simulink model "ScriptDemo"  (R2022b)
settings: configuration reference "TmVcThermal_Configuration_sub" (kept outside this file)
undefined symbols (not defined in the file): aaaa, bbbb, cTmComprCtrl_D_u8HvacFlowTable_db, cTmComprCtrl_D_u8HvacFlowTable_sw, cTmComprCtrl_n_i16ChillCmpIMax, cTmComprCtrl_n_i16ChillCmpIMin, cTmComprCtrl_n_i16ChillCmpIMin666, cTmComprCtrl_n_i16ChillCmpPMax, cTmComprCtrl_n_i16ChillCmpPMin, cTmComprCtrl_n_i16CmpChillCoolRpmKiMax, cTmComprCtrl_n_i16CmpChillCoolRpmKiMin, cTmComprCtrl_n_i16CmpChillCoolRpmKpMax, cTmComprCtrl_n_i16CmpChillCoolRpmKpMin, cTmComprCtrl_n_i16CmpCoolRpmKiMax, cTmComprCtrl_n_i16CmpCoolRpmKiMin, cTmComprCtrl_n_i16CmpCoolRpmKpMax, cTmComprCtrl_n_i16CmpCoolRpmKpMin, cTmComprCtrl_n_i16SM4CmpHeatKiMax, cTmComprCtrl_n_i16SM4CmpHeatKiMin, cTmComprCtrl_n_i16SM4CmpHeatKpMax, cTmComprCtrl_n_i16SM4CmpHeatKpMin, cTmComprCtrl_n_i16SM5CmpHeatKiMax, cTmComprCtrl_n_i16SM5CmpHeatKiMin, cTmComprCtrl_n_i16SM5CmpHeatKpMax, cTmComprCtrl_n_i16SM5CmpHeatKpMin, cTmComprCtrl_n_i16SM6CmpHeatKiMax, cTmComprCtrl_n_i16SM6CmpHeatKiMin, cTmComprCtrl_n_i16SM6CmpHeatKpMax, cTmComprCtrl_n_i16SM6CmpHeatKpMin, cTmComprCtrl_n_u16CmpMaxSpdFanFltLimt, cTmComprCtrl_n_u16CmpMaxSpdLoSidePFltLimt, cTmComprCtrl_n_u16CmpMaxSpdSensorFltLimt, cTmComprCtrl_n_u16CompMinRpm, cTmComprCtrl_n_u16CompRpmIncThres, cTmComprCtrl_t_u16BattCooltFFPeriod, cTmComprCtrl_t_u16BattCooltPIPeriod, cTmComprCtrl_t_u16CmpCoolFFPeriod, cTmComprCtrl_t_u16CmpCoolPIPeriod, cTmComprCtrl_t_u16CoolCmpChillFFPeriod, cTmComprCtrl_t_u16CoolCmpChillPIPeriod, cTmComprCtrl_t_u16SM4CmpHeatFFPeriod, cTmComprCtrl_t_u16SM4CmpHeatPIPeriod, cTmComprCtrl_t_u16SM5CmpHeatFFPeriod, cTmComprCtrl_t_u16SM5CmpHeatPIPeriod, cTmComprCtrl_t_u16SM6CmpHeatFFPeriod, cTmComprCtrl_t_u16SM6CmpHeatPIPeriod, cTmComprCtrl_Te_EvapClearInteg, cTmComprCtrl_Te_i16HpReqTempSaturoffset, cTmComprCtrl_Te_i16SatLpReplaceDiff, cTmComprCtrl_Te_i16SM3BatDiffStartEvapDecOffset, cTmComprCtrl_Te_i16SM3EvapLo, cTmComprCtrl_Te_i16SM3TBatDiffEntEvapDecOffset, cTmComprCtrl_Te_i16SM3TBatDiffEntEvapDecOffsetQuit, cTmComprCtrl_Te_s32ErrCmpChillPIContinueCoolH, cTmComprCtrl_Te_s32ErrCmpChillPIContinueCoolL, cTmComprCtrl_Te_s32ErrCmpPIContinueChillH, cTmComprCtrl_Te_s32ErrCmpPIContinueChillL, cTmComprCtrl_Te_s32ErrCmpPIContinueCoolH, cTmComprCtrl_Te_s32ErrCmpPIContinueCoolL, cTmComprCtrl_Te_s32ErrCmpPIContinueHeatH ... (+398)
libraries: simulink x782, PCMULib x640, simulink_need_slupdate x4
(part 10 of 41)

== system ScriptDemo/Create/Model/createModSig/After3 ==
  note: % 鼠标选中模型执行如下代码
      | createModSig(gcb,' testValue ',true)
  sTmRefriVlvCtrl_X_s32CEXVPosReqIn : Inport  OutDataTypeStr=single  OutputFunctionCall=on
  sTmRefriVlvCtrl_X_s32EEXVPosReqIn : Inport  Port=2  OutDataTypeStr=single
  sTmRefriVlvCtrl_X_s32BEXVPosReqIn : Inport  Port=3  OutDataTypeStr=single
  yTmRefriVlvCtrl_B_HpcCexvMovEnableIn : Inport  Port=4  OutDataTypeStr=boolean
  sTmRefriVlvCtrl_Z_u8CEXVInitStateIn : Inport  Port=5  OutDataTypeStr=uint8
  yTmRefriVlvCtrl_B_CexvCalibReqIn : Inport  Port=6  OutDataTypeStr=boolean
  yTmRefriVlvCtrl_B_HpcEexvMovEnableIn : Inport  Port=7  OutDataTypeStr=boolean
  sTmRefriVlvCtrl_Z_u8EEXVInitStateIn : Inport  Port=8  OutDataTypeStr=uint8
  yTmRefriVlvCtrl_B_EexvCalibReqIn : Inport  Port=9  OutDataTypeStr=boolean
  yTmRefriVlvCtrl_B_HpcBexvMovEnableIn : Inport  Port=10  OutDataTypeStr=boolean
  sTmRefriVlvCtrl_Z_u8BEXVInitStateIn : Inport  Port=11  OutDataTypeStr=uint8
  yTmRefriVlvCtrl_B_BexvCalibReqIn : Inport  Port=12  OutDataTypeStr=boolean
  sTmRefriVlvCtrl_X_s32SM3BexvMaxPosIn : Inport  Port=13  OutDataTypeStr=single
  yTmRefriVlvCtrl_B_EvapBattTLimBexvEnaIn : Inport  Port=14  OutDataTypeStr=boolean
  sTmRefriVlvCtrl_D_u8EexvRefriSwitchStIn : Inport  Port=15  OutDataTypeStr=uint8
  sTmRefriVlvCtrl_D_u8CexvRefriSwitchStIn : Inport  Port=16  OutDataTypeStr=uint8
  sTmRefriVlvCtrl_D_u8BexvRefriSwitchStIn : Inport  Port=17  OutDataTypeStr=uint8
  Before : Subsystem
  sTmRefriVlvCtrl_X_s32CEXVPosReq : Outport  OutDataTypeStr=single
  sTmRefriVlvCtrl_X_s32EEXVPosReq : Outport  Port=2  OutDataTypeStr=single
  sTmRefriVlvCtrl_X_s32BEXVPosReq : Outport  Port=3  OutDataTypeStr=single
  yTmRefriVlvCtrl_B_HpcCexvMovEnable : Outport  Port=4  OutDataTypeStr=boolean
  sTmRefriVlvCtrl_Z_u8CEXVInitState : Outport  Port=5  OutDataTypeStr=uint8
  yTmRefriVlvCtrl_B_CexvCalibReq : Outport  Port=6  OutDataTypeStr=boolean
  yTmRefriVlvCtrl_B_HpcEexvMovEnable : Outport  Port=7  OutDataTypeStr=boolean
  sTmRefriVlvCtrl_Z_u8EEXVInitState : Outport  Port=8  OutDataTypeStr=uint8
  yTmRefriVlvCtrl_B_EexvCalibReq : Outport  Port=9  OutDataTypeStr=boolean
  yTmRefriVlvCtrl_B_HpcBexvMovEnable : Outport  Port=10  OutDataTypeStr=boolean
  sTmRefriVlvCtrl_Z_u8BEXVInitState : Outport  Port=11  OutDataTypeStr=uint8
  yTmRefriVlvCtrl_B_BexvCalibReq : Outport  Port=12  OutDataTypeStr=boolean
  sTmRefriVlvCtrl_X_s32SM3BexvMaxPos : Outport  Port=13  OutDataTypeStr=single
  yTmRefriVlvCtrl_B_EvapBattTLimBexvEna : Outport  Port=14  OutDataTypeStr=boolean
  sTmRefriVlvCtrl_D_u8EexvRefriSwitchSt : Outport  Port=15  OutDataTypeStr=uint8
  sTmRefriVlvCtrl_D_u8CexvRefriSwitchSt : Outport  Port=16  OutDataTypeStr=uint8
  sTmRefriVlvCtrl_D_u8BexvRefriSwitchSt : Outport  Port=17  OutDataTypeStr=uint8
  wires:
  sTmRefriVlvCtrl_X_s32BEXVPosReqIn/1 -> Before/3(sTmRefriVlvCtrl_X_s32BEXVPosReqIn)  "sTmRefriVlvCtrl_X_s32BEXVPosReqIn"
  sTmRefriVlvCtrl_X_s32SM3BexvMaxPosIn/1 -> Before/13(sTmRefriVlvCtrl_X_s32SM3BexvMaxPosIn)  "sTmRefriVlvCtrl_X_s32SM3BexvMaxPosIn"
  sTmRefriVlvCtrl_Z_u8BEXVInitStateIn/1 -> Before/11(sTmRefriVlvCtrl_Z_u8BEXVInitStateIn)  "sTmRefriVlvCtrl_Z_u8BEXVInitStateIn"
  sTmRefriVlvCtrl_D_u8CexvRefriSwitchStIn/1 -> Before/16(sTmRefriVlvCtrl_D_u8CexvRefriSwitchStIn)  "sTmRefriVlvCtrl_D_u8CexvRefriSwitchStIn"
  yTmRefriVlvCtrl_B_EvapBattTLimBexvEnaIn/1 -> Before/14(yTmRefriVlvCtrl_B_EvapBattTLimBexvEnaIn)  "yTmRefriVlvCtrl_B_EvapBattTLimBexvEnaIn"
  yTmRefriVlvCtrl_B_HpcEexvMovEnableIn/1 -> Before/7(yTmRefriVlvCtrl_B_HpcEexvMovEnableIn)  "yTmRefriVlvCtrl_B_HpcEexvMovEnableIn"
  Before/3(sTmRefriVlvCtrl_X_s32BEXVPosReq) -> sTmRefriVlvCtrl_X_s32BEXVPosReq/1  "sTmRefriVlvCtrl_X_s32BEXVPosReq"
  yTmRefriVlvCtrl_B_EexvCalibReqIn/1 -> Before/9(yTmRefriVlvCtrl_B_EexvCalibReqIn)  "yTmRefriVlvCtrl_B_EexvCalibReqIn"
  Before/8(sTmRefriVlvCtrl_Z_u8EEXVInitState) -> sTmRefriVlvCtrl_Z_u8EEXVInitState/1  "sTmRefriVlvCtrl_Z_u8EEXVInitState"
  sTmRefriVlvCtrl_Z_u8EEXVInitStateIn/1 -> Before/8(sTmRefriVlvCtrl_Z_u8EEXVInitStateIn)  "sTmRefriVlvCtrl_Z_u8EEXVInitStateIn"
  yTmRefriVlvCtrl_B_HpcBexvMovEnableIn/1 -> Before/10(yTmRefriVlvCtrl_B_HpcBexvMovEnableIn)  "yTmRefriVlvCtrl_B_HpcBexvMovEnableIn"
  yTmRefriVlvCtrl_B_BexvCalibReqIn/1 -> Before/12(yTmRefriVlvCtrl_B_BexvCalibReqIn)  "yTmRefriVlvCtrl_B_BexvCalibReqIn"
  Before/5(sTmRefriVlvCtrl_Z_u8CEXVInitState) -> sTmRefriVlvCtrl_Z_u8CEXVInitState/1  "sTmRefriVlvCtrl_Z_u8CEXVInitState"
  Before/4(yTmRefriVlvCtrl_B_HpcCexvMovEnable) -> yTmRefriVlvCtrl_B_HpcCexvMovEnable/1  "yTmRefriVlvCtrl_B_HpcCexvMovEnable"
  Before/6(yTmRefriVlvCtrl_B_CexvCalibReq) -> yTmRefriVlvCtrl_B_CexvCalibReq/1  "yTmRefriVlvCtrl_B_CexvCalibReq"
  sTmRefriVlvCtrl_X_s32EEXVPosReqIn/1 -> Before/2(sTmRefriVlvCtrl_X_s32EEXVPosReqIn)  "sTmRefriVlvCtrl_X_s32EEXVPosReqIn"
  sTmRefriVlvCtrl_X_s32CEXVPosReqIn/1 -> Before/1(sTmRefriVlvCtrl_X_s32CEXVPosReqIn)  "sTmRefriVlvCtrl_X_s32CEXVPosReqIn"
  yTmRefriVlvCtrl_B_CexvCalibReqIn/1 -> Before/6(yTmRefriVlvCtrl_B_CexvCalibReqIn)  "yTmRefriVlvCtrl_B_CexvCalibReqIn"
  sTmRefriVlvCtrl_Z_u8CEXVInitStateIn/1 -> Before/5(sTmRefriVlvCtrl_Z_u8CEXVInitStateIn)  "sTmRefriVlvCtrl_Z_u8CEXVInitStateIn"
  yTmRefriVlvCtrl_B_HpcCexvMovEnableIn/1 -> Before/4(yTmRefriVlvCtrl_B_HpcCexvMovEnableIn)  "yTmRefriVlvCtrl_B_HpcCexvMovEnableIn"
  sTmRefriVlvCtrl_D_u8BexvRefriSwitchStIn/1 -> Before/17(sTmRefriVlvCtrl_D_u8BexvRefriSwitchStIn)  "sTmRefriVlvCtrl_D_u8BexvRefriSwitchStIn"
  Before/12(yTmRefriVlvCtrl_B_BexvCalibReq) -> yTmRefriVlvCtrl_B_BexvCalibReq/1  "yTmRefriVlvCtrl_B_BexvCalibReq"
  Before/11(sTmRefriVlvCtrl_Z_u8BEXVInitState) -> sTmRefriVlvCtrl_Z_u8BEXVInitState/1  "sTmRefriVlvCtrl_Z_u8BEXVInitState"
  Before/1(sTmRefriVlvCtrl_X_s32CEXVPosReq) -> sTmRefriVlvCtrl_X_s32CEXVPosReq/1  "sTmRefriVlvCtrl_X_s32CEXVPosReq"
  Before/7(yTmRefriVlvCtrl_B_HpcEexvMovEnable) -> yTmRefriVlvCtrl_B_HpcEexvMovEnable/1  "yTmRefriVlvCtrl_B_HpcEexvMovEnable"
  sTmRefriVlvCtrl_D_u8EexvRefriSwitchStIn/1 -> Before/15(sTmRefriVlvCtrl_D_u8EexvRefriSwitchStIn)  "sTmRefriVlvCtrl_D_u8EexvRefriSwitchStIn"
  Before/10(yTmRefriVlvCtrl_B_HpcBexvMovEnable) -> yTmRefriVlvCtrl_B_HpcBexvMovEnable/1  "yTmRefriVlvCtrl_B_HpcBexvMovEnable"
  Before/14(yTmRefriVlvCtrl_B_EvapBattTLimBexvEna) -> yTmRefriVlvCtrl_B_EvapBattTLimBexvEna/1  "yTmRefriVlvCtrl_B_EvapBattTLimBexvEna"
  Before/9(yTmRefriVlvCtrl_B_EexvCalibReq) -> yTmRefriVlvCtrl_B_EexvCalibReq/1  "yTmRefriVlvCtrl_B_EexvCalibReq"
  Before/15(sTmRefriVlvCtrl_D_u8EexvRefriSwitchSt) -> sTmRefriVlvCtrl_D_u8EexvRefriSwitchSt/1  "sTmRefriVlvCtrl_D_u8EexvRefriSwitchSt"
  Before/13(sTmRefriVlvCtrl_X_s32SM3BexvMaxPos) -> sTmRefriVlvCtrl_X_s32SM3BexvMaxPos/1  "sTmRefriVlvCtrl_X_s32SM3BexvMaxPos"
  Before/17(sTmRefriVlvCtrl_D_u8BexvRefriSwitchSt) -> sTmRefriVlvCtrl_D_u8BexvRefriSwitchSt/1  "sTmRefriVlvCtrl_D_u8BexvRefriSwitchSt"
  Before/2(sTmRefriVlvCtrl_X_s32EEXVPosReq) -> sTmRefriVlvCtrl_X_s32EEXVPosReq/1  "sTmRefriVlvCtrl_X_s32EEXVPosReq"
  Before/16(sTmRefriVlvCtrl_D_u8CexvRefriSwitchSt) -> sTmRefriVlvCtrl_D_u8CexvRefriSwitchSt/1  "sTmRefriVlvCtrl_D_u8CexvRefriSwitchSt"

== system ScriptDemo/Create/Model/createModSig/After4 ==
  note: % 鼠标选中模型执行如下代码
      | createModSig(gcb,' dispName ',true)
  sTmRefriVlvCtrl_X_s32CEXVPosReqIn : Inport  OutDataTypeStr=single  OutputFunctionCall=on
  sTmRefriVlvCtrl_X_s32EEXVPosReqIn : Inport  Port=2  OutDataTypeStr=single
  sTmRefriVlvCtrl_X_s32BEXVPosReqIn : Inport  Port=3  OutDataTypeStr=single
  yTmRefriVlvCtrl_B_HpcCexvMovEnableIn : Inport  Port=4  OutDataTypeStr=boolean
  sTmRefriVlvCtrl_Z_u8CEXVInitStateIn : Inport  Port=5  OutDataTypeStr=uint8
  yTmRefriVlvCtrl_B_CexvCalibReqIn : Inport  Port=6  OutDataTypeStr=boolean
  yTmRefriVlvCtrl_B_HpcEexvMovEnableIn : Inport  Port=7  OutDataTypeStr=boolean
  sTmRefriVlvCtrl_Z_u8EEXVInitStateIn : Inport  Port=8  OutDataTypeStr=uint8
  yTmRefriVlvCtrl_B_EexvCalibReqIn : Inport  Port=9  OutDataTypeStr=boolean
  yTmRefriVlvCtrl_B_HpcBexvMovEnableIn : Inport  Port=10  OutDataTypeStr=boolean
  sTmRefriVlvCtrl_Z_u8BEXVInitStateIn : Inport  Port=11  OutDataTypeStr=uint8
  yTmRefriVlvCtrl_B_BexvCalibReqIn : Inport  Port=12  OutDataTypeStr=boolean
  sTmRefriVlvCtrl_X_s32SM3BexvMaxPosIn : Inport  Port=13  OutDataTypeStr=single
  yTmRefriVlvCtrl_B_EvapBattTLimBexvEnaIn : Inport  Port=14  OutDataTypeStr=boolean
  sTmRefriVlvCtrl_D_u8EexvRefriSwitchStIn : Inport  Port=15  OutDataTypeStr=uint8
  sTmRefriVlvCtrl_D_u8CexvRefriSwitchStIn : Inport  Port=16  OutDataTypeStr=uint8
  sTmRefriVlvCtrl_D_u8BexvRefriSwitchStIn : Inport  Port=17  OutDataTypeStr=uint8
  Before : Subsystem
  sTmRefriVlvCtrl_X_s32CEXVPosReq : Outport  OutDataTypeStr=single
  sTmRefriVlvCtrl_X_s32EEXVPosReq : Outport  Port=2  OutDataTypeStr=single
  sTmRefriVlvCtrl_X_s32BEXVPosReq : Outport  Port=3  OutDataTypeStr=single
  yTmRefriVlvCtrl_B_HpcCexvMovEnable : Outport  Port=4  OutDataTypeStr=boolean
  sTmRefriVlvCtrl_Z_u8CEXVInitState : Outport  Port=5  OutDataTypeStr=uint8
  yTmRefriVlvCtrl_B_CexvCalibReq : Outport  Port=6  OutDataTypeStr=boolean
  yTmRefriVlvCtrl_B_HpcEexvMovEnable : Outport  Port=7  OutDataTypeStr=boolean
  sTmRefriVlvCtrl_Z_u8EEXVInitState : Outport  Port=8  OutDataTypeStr=uint8
  yTmRefriVlvCtrl_B_EexvCalibReq : Outport  Port=9  OutDataTypeStr=boolean
  yTmRefriVlvCtrl_B_HpcBexvMovEnable : Outport  Port=10  OutDataTypeStr=boolean
  sTmRefriVlvCtrl_Z_u8BEXVInitState : Outport  Port=11  OutDataTypeStr=uint8
  yTmRefriVlvCtrl_B_BexvCalibReq : Outport  Port=12  OutDataTypeStr=boolean
  sTmRefriVlvCtrl_X_s32SM3BexvMaxPos : Outport  Port=13  OutDataTypeStr=single
  yTmRefriVlvCtrl_B_EvapBattTLimBexvEna : Outport  Port=14  OutDataTypeStr=boolean
  sTmRefriVlvCtrl_D_u8EexvRefriSwitchSt : Outport  Port=15  OutDataTypeStr=uint8
  sTmRefriVlvCtrl_D_u8CexvRefriSwitchSt : Outport  Port=16  OutDataTypeStr=uint8
  sTmRefriVlvCtrl_D_u8BexvRefriSwitchSt : Outport  Port=17  OutDataTypeStr=uint8
  wires:
  sTmRefriVlvCtrl_X_s32BEXVPosReqIn/1 -> Before/3(sTmRefriVlvCtrl_X_s32BEXVPosReqIn)  "sTmRefriVlvCtrl_X_s32BEXVPosReqIn"
  sTmRefriVlvCtrl_X_s32SM3BexvMaxPosIn/1 -> Before/13(sTmRefriVlvCtrl_X_s32SM3BexvMaxPosIn)  "sTmRefriVlvCtrl_X_s32SM3BexvMaxPosIn"
  sTmRefriVlvCtrl_Z_u8BEXVInitStateIn/1 -> Before/11(sTmRefriVlvCtrl_Z_u8BEXVInitStateIn)  "sTmRefriVlvCtrl_Z_u8BEXVInitStateIn"
  sTmRefriVlvCtrl_D_u8CexvRefriSwitchStIn/1 -> Before/16(sTmRefriVlvCtrl_D_u8CexvRefriSwitchStIn)  "sTmRefriVlvCtrl_D_u8CexvRefriSwitchStIn"
  yTmRefriVlvCtrl_B_EvapBattTLimBexvEnaIn/1 -> Before/14(yTmRefriVlvCtrl_B_EvapBattTLimBexvEnaIn)  "yTmRefriVlvCtrl_B_EvapBattTLimBexvEnaIn"
  yTmRefriVlvCtrl_B_HpcEexvMovEnableIn/1 -> Before/7(yTmRefriVlvCtrl_B_HpcEexvMovEnableIn)  "yTmRefriVlvCtrl_B_HpcEexvMovEnableIn"
  Before/3(sTmRefriVlvCtrl_X_s32BEXVPosReq) -> sTmRefriVlvCtrl_X_s32BEXVPosReq/1  "sTmRefriVlvCtrl_X_s32BEXVPosReq"
  yTmRefriVlvCtrl_B_EexvCalibReqIn/1 -> Before/9(yTmRefriVlvCtrl_B_EexvCalibReqIn)  "yTmRefriVlvCtrl_B_EexvCalibReqIn"
  Before/8(sTmRefriVlvCtrl_Z_u8EEXVInitState) -> sTmRefriVlvCtrl_Z_u8EEXVInitState/1  "sTmRefriVlvCtrl_Z_u8EEXVInitState"
  sTmRefriVlvCtrl_Z_u8EEXVInitStateIn/1 -> Before/8(sTmRefriVlvCtrl_Z_u8EEXVInitStateIn)  "sTmRefriVlvCtrl_Z_u8EEXVInitStateIn"
  yTmRefriVlvCtrl_B_HpcBexvMovEnableIn/1 -> Before/10(yTmRefriVlvCtrl_B_HpcBexvMovEnableIn)  "yTmRefriVlvCtrl_B_HpcBexvMovEnableIn"
  yTmRefriVlvCtrl_B_BexvCalibReqIn/1 -> Before/12(yTmRefriVlvCtrl_B_BexvCalibReqIn)  "yTmRefriVlvCtrl_B_BexvCalibReqIn"
  Before/5(sTmRefriVlvCtrl_Z_u8CEXVInitState) -> sTmRefriVlvCtrl_Z_u8CEXVInitState/1  "sTmRefriVlvCtrl_Z_u8CEXVInitState"
  Before/4(yTmRefriVlvCtrl_B_HpcCexvMovEnable) -> yTmRefriVlvCtrl_B_HpcCexvMovEnable/1  "yTmRefriVlvCtrl_B_HpcCexvMovEnable"
  Before/6(yTmRefriVlvCtrl_B_CexvCalibReq) -> yTmRefriVlvCtrl_B_CexvCalibReq/1  "yTmRefriVlvCtrl_B_CexvCalibReq"
  sTmRefriVlvCtrl_X_s32EEXVPosReqIn/1 -> Before/2(sTmRefriVlvCtrl_X_s32EEXVPosReqIn)  "sTmRefriVlvCtrl_X_s32EEXVPosReqIn"
  sTmRefriVlvCtrl_X_s32CEXVPosReqIn/1 -> Before/1(sTmRefriVlvCtrl_X_s32CEXVPosReqIn)  "sTmRefriVlvCtrl_X_s32CEXVPosReqIn"
  yTmRefriVlvCtrl_B_CexvCalibReqIn/1 -> Before/6(yTmRefriVlvCtrl_B_CexvCalibReqIn)  "yTmRefriVlvCtrl_B_CexvCalibReqIn"
  sTmRefriVlvCtrl_Z_u8CEXVInitStateIn/1 -> Before/5(sTmRefriVlvCtrl_Z_u8CEXVInitStateIn)  "sTmRefriVlvCtrl_Z_u8CEXVInitStateIn"
  yTmRefriVlvCtrl_B_HpcCexvMovEnableIn/1 -> Before/4(yTmRefriVlvCtrl_B_HpcCexvMovEnableIn)  "yTmRefriVlvCtrl_B_HpcCexvMovEnableIn"
  sTmRefriVlvCtrl_D_u8BexvRefriSwitchStIn/1 -> Before/17(sTmRefriVlvCtrl_D_u8BexvRefriSwitchStIn)  "sTmRefriVlvCtrl_D_u8BexvRefriSwitchStIn"
  Before/12(yTmRefriVlvCtrl_B_BexvCalibReq) -> yTmRefriVlvCtrl_B_BexvCalibReq/1  "yTmRefriVlvCtrl_B_BexvCalibReq"
  Before/11(sTmRefriVlvCtrl_Z_u8BEXVInitState) -> sTmRefriVlvCtrl_Z_u8BEXVInitState/1  "sTmRefriVlvCtrl_Z_u8BEXVInitState"
  Before/1(sTmRefriVlvCtrl_X_s32CEXVPosReq) -> sTmRefriVlvCtrl_X_s32CEXVPosReq/1  "sTmRefriVlvCtrl_X_s32CEXVPosReq"
  Before/7(yTmRefriVlvCtrl_B_HpcEexvMovEnable) -> yTmRefriVlvCtrl_B_HpcEexvMovEnable/1  "yTmRefriVlvCtrl_B_HpcEexvMovEnable"
  sTmRefriVlvCtrl_D_u8EexvRefriSwitchStIn/1 -> Before/15(sTmRefriVlvCtrl_D_u8EexvRefriSwitchStIn)  "sTmRefriVlvCtrl_D_u8EexvRefriSwitchStIn"
  Before/10(yTmRefriVlvCtrl_B_HpcBexvMovEnable) -> yTmRefriVlvCtrl_B_HpcBexvMovEnable/1  "yTmRefriVlvCtrl_B_HpcBexvMovEnable"
  Before/14(yTmRefriVlvCtrl_B_EvapBattTLimBexvEna) -> yTmRefriVlvCtrl_B_EvapBattTLimBexvEna/1  "yTmRefriVlvCtrl_B_EvapBattTLimBexvEna"
  Before/9(yTmRefriVlvCtrl_B_EexvCalibReq) -> yTmRefriVlvCtrl_B_EexvCalibReq/1  "yTmRefriVlvCtrl_B_EexvCalibReq"
  Before/15(sTmRefriVlvCtrl_D_u8EexvRefriSwitchSt) -> sTmRefriVlvCtrl_D_u8EexvRefriSwitchSt/1  "sTmRefriVlvCtrl_D_u8EexvRefriSwitchSt"
  Before/13(sTmRefriVlvCtrl_X_s32SM3BexvMaxPos) -> sTmRefriVlvCtrl_X_s32SM3BexvMaxPos/1  "sTmRefriVlvCtrl_X_s32SM3BexvMaxPos"
  Before/17(sTmRefriVlvCtrl_D_u8BexvRefriSwitchSt) -> sTmRefriVlvCtrl_D_u8BexvRefriSwitchSt/1  "sTmRefriVlvCtrl_D_u8BexvRefriSwitchSt"
  Before/2(sTmRefriVlvCtrl_X_s32EEXVPosReq) -> sTmRefriVlvCtrl_X_s32EEXVPosReq/1  "sTmRefriVlvCtrl_X_s32EEXVPosReq"
  Before/16(sTmRefriVlvCtrl_D_u8CexvRefriSwitchSt) -> sTmRefriVlvCtrl_D_u8CexvRefriSwitchSt/1  "sTmRefriVlvCtrl_D_u8CexvRefriSwitchSt"

== system ScriptDemo/Create/Model/createModSig/Before ==
  sTmRefriVlvCtrl_X_s32CEXVPosReqIn : Inport  OutDataTypeStr=single  OutputFunctionCall=on
  sTmRefriVlvCtrl_X_s32EEXVPosReqIn : Inport  Port=2  OutDataTypeStr=single
  sTmRefriVlvCtrl_X_s32BEXVPosReqIn : Inport  Port=3  OutDataTypeStr=single
  yTmRefriVlvCtrl_B_HpcCexvMovEnableIn : Inport  Port=4  OutDataTypeStr=boolean
  sTmRefriVlvCtrl_Z_u8CEXVInitStateIn : Inport  Port=5  OutDataTypeStr=uint8
  yTmRefriVlvCtrl_B_CexvCalibReqIn : Inport  Port=6  OutDataTypeStr=boolean
  yTmRefriVlvCtrl_B_HpcEexvMovEnableIn : Inport  Port=7  OutDataTypeStr=boolean
  sTmRefriVlvCtrl_Z_u8EEXVInitStateIn : Inport  Port=8  OutDataTypeStr=uint8
  yTmRefriVlvCtrl_B_EexvCalibReqIn : Inport  Port=9  OutDataTypeStr=boolean
  yTmRefriVlvCtrl_B_HpcBexvMovEnableIn : Inport  Port=10  OutDataTypeStr=boolean
  sTmRefriVlvCtrl_Z_u8BEXVInitStateIn : Inport  Port=11  OutDataTypeStr=uint8
  yTmRefriVlvCtrl_B_BexvCalibReqIn : Inport  Port=12  OutDataTypeStr=boolean
  sTmRefriVlvCtrl_X_s32SM3BexvMaxPosIn : Inport  Port=13  OutDataTypeStr=single
  yTmRefriVlvCtrl_B_EvapBattTLimBexvEnaIn : Inport  Port=14  OutDataTypeStr=boolean
  sTmRefriVlvCtrl_D_u8EexvRefriSwitchStIn : Inport  Port=15  OutDataTypeStr=uint8
  sTmRefriVlvCtrl_D_u8CexvRefriSwitchStIn : Inport  Port=16  OutDataTypeStr=uint8
  sTmRefriVlvCtrl_D_u8BexvRefriSwitchStIn : Inport  Port=17  OutDataTypeStr=uint8
  Before : Subsystem
  sTmRefriVlvCtrl_X_s32CEXVPosReq : Outport  OutDataTypeStr=single
  sTmRefriVlvCtrl_X_s32EEXVPosReq : Outport  Port=2  OutDataTypeStr=single
  sTmRefriVlvCtrl_X_s32BEXVPosReq : Outport  Port=3  OutDataTypeStr=single
  yTmRefriVlvCtrl_B_HpcCexvMovEnable : Outport  Port=4  OutDataTypeStr=boolean
  sTmRefriVlvCtrl_Z_u8CEXVInitState : Outport  Port=5  OutDataTypeStr=uint8
  yTmRefriVlvCtrl_B_CexvCalibReq : Outport  Port=6  OutDataTypeStr=boolean
  yTmRefriVlvCtrl_B_HpcEexvMovEnable : Outport  Port=7  OutDataTypeStr=boolean
  sTmRefriVlvCtrl_Z_u8EEXVInitState : Outport  Port=8  OutDataTypeStr=uint8
  yTmRefriVlvCtrl_B_EexvCalibReq : Outport  Port=9  OutDataTypeStr=boolean
  yTmRefriVlvCtrl_B_HpcBexvMovEnable : Outport  Port=10  OutDataTypeStr=boolean
  sTmRefriVlvCtrl_Z_u8BEXVInitState : Outport  Port=11  OutDataTypeStr=uint8
  yTmRefriVlvCtrl_B_BexvCalibReq : Outport  Port=12  OutDataTypeStr=boolean
  sTmRefriVlvCtrl_X_s32SM3BexvMaxPos : Outport  Port=13  OutDataTypeStr=single
  yTmRefriVlvCtrl_B_EvapBattTLimBexvEna : Outport  Port=14  OutDataTypeStr=boolean
  sTmRefriVlvCtrl_D_u8EexvRefriSwitchSt : Outport  Port=15  OutDataTypeStr=uint8
  sTmRefriVlvCtrl_D_u8CexvRefriSwitchSt : Outport  Port=16  OutDataTypeStr=uint8
  sTmRefriVlvCtrl_D_u8BexvRefriSwitchSt : Outport  Port=17  OutDataTypeStr=uint8
  wires:
  sTmRefriVlvCtrl_X_s32CEXVPosReqIn/1 -> Before/1(sTmRefriVlvCtrl_X_s32CEXVPosReqIn)
  sTmRefriVlvCtrl_X_s32EEXVPosReqIn/1 -> Before/2(sTmRefriVlvCtrl_X_s32EEXVPosReqIn)
  sTmRefriVlvCtrl_X_s32BEXVPosReqIn/1 -> Before/3(sTmRefriVlvCtrl_X_s32BEXVPosReqIn)
  yTmRefriVlvCtrl_B_HpcCexvMovEnableIn/1 -> Before/4(yTmRefriVlvCtrl_B_HpcCexvMovEnableIn)
  sTmRefriVlvCtrl_Z_u8CEXVInitStateIn/1 -> Before/5(sTmRefriVlvCtrl_Z_u8CEXVInitStateIn)
  yTmRefriVlvCtrl_B_CexvCalibReqIn/1 -> Before/6(yTmRefriVlvCtrl_B_CexvCalibReqIn)
  yTmRefriVlvCtrl_B_HpcEexvMovEnableIn/1 -> Before/7(yTmRefriVlvCtrl_B_HpcEexvMovEnableIn)
  sTmRefriVlvCtrl_Z_u8EEXVInitStateIn/1 -> Before/8(sTmRefriVlvCtrl_Z_u8EEXVInitStateIn)
  yTmRefriVlvCtrl_B_EexvCalibReqIn/1 -> Before/9(yTmRefriVlvCtrl_B_EexvCalibReqIn)
  yTmRefriVlvCtrl_B_HpcBexvMovEnableIn/1 -> Before/10(yTmRefriVlvCtrl_B_HpcBexvMovEnableIn)
  sTmRefriVlvCtrl_Z_u8BEXVInitStateIn/1 -> Before/11(sTmRefriVlvCtrl_Z_u8BEXVInitStateIn)
  yTmRefriVlvCtrl_B_BexvCalibReqIn/1 -> Before/12(yTmRefriVlvCtrl_B_BexvCalibReqIn)
  sTmRefriVlvCtrl_X_s32SM3BexvMaxPosIn/1 -> Before/13(sTmRefriVlvCtrl_X_s32SM3BexvMaxPosIn)
  yTmRefriVlvCtrl_B_EvapBattTLimBexvEnaIn/1 -> Before/14(yTmRefriVlvCtrl_B_EvapBattTLimBexvEnaIn)
  sTmRefriVlvCtrl_D_u8EexvRefriSwitchStIn/1 -> Before/15(sTmRefriVlvCtrl_D_u8EexvRefriSwitchStIn)
  sTmRefriVlvCtrl_D_u8CexvRefriSwitchStIn/1 -> Before/16(sTmRefriVlvCtrl_D_u8CexvRefriSwitchStIn)
  sTmRefriVlvCtrl_D_u8BexvRefriSwitchStIn/1 -> Before/17(sTmRefriVlvCtrl_D_u8BexvRefriSwitchStIn)
  Before/1(sTmRefriVlvCtrl_X_s32CEXVPosReq) -> sTmRefriVlvCtrl_X_s32CEXVPosReq/1
  Before/2(sTmRefriVlvCtrl_X_s32EEXVPosReq) -> sTmRefriVlvCtrl_X_s32EEXVPosReq/1
  Before/3(sTmRefriVlvCtrl_X_s32BEXVPosReq) -> sTmRefriVlvCtrl_X_s32BEXVPosReq/1
  Before/4(yTmRefriVlvCtrl_B_HpcCexvMovEnable) -> yTmRefriVlvCtrl_B_HpcCexvMovEnable/1
  Before/5(sTmRefriVlvCtrl_Z_u8CEXVInitState) -> sTmRefriVlvCtrl_Z_u8CEXVInitState/1
  Before/6(yTmRefriVlvCtrl_B_CexvCalibReq) -> yTmRefriVlvCtrl_B_CexvCalibReq/1
  Before/7(yTmRefriVlvCtrl_B_HpcEexvMovEnable) -> yTmRefriVlvCtrl_B_HpcEexvMovEnable/1
  Before/8(sTmRefriVlvCtrl_Z_u8EEXVInitState) -> sTmRefriVlvCtrl_Z_u8EEXVInitState/1
  Before/9(yTmRefriVlvCtrl_B_EexvCalibReq) -> yTmRefriVlvCtrl_B_EexvCalibReq/1
  Before/10(yTmRefriVlvCtrl_B_HpcBexvMovEnable) -> yTmRefriVlvCtrl_B_HpcBexvMovEnable/1
  Before/11(sTmRefriVlvCtrl_Z_u8BEXVInitState) -> sTmRefriVlvCtrl_Z_u8BEXVInitState/1
  Before/12(yTmRefriVlvCtrl_B_BexvCalibReq) -> yTmRefriVlvCtrl_B_BexvCalibReq/1
  Before/13(sTmRefriVlvCtrl_X_s32SM3BexvMaxPos) -> sTmRefriVlvCtrl_X_s32SM3BexvMaxPos/1
  Before/14(yTmRefriVlvCtrl_B_EvapBattTLimBexvEna) -> yTmRefriVlvCtrl_B_EvapBattTLimBexvEna/1
  Before/15(sTmRefriVlvCtrl_D_u8EexvRefriSwitchSt) -> sTmRefriVlvCtrl_D_u8EexvRefriSwitchSt/1
  Before/16(sTmRefriVlvCtrl_D_u8CexvRefriSwitchSt) -> sTmRefriVlvCtrl_D_u8CexvRefriSwitchSt/1
  Before/17(sTmRefriVlvCtrl_D_u8BexvRefriSwitchSt) -> sTmRefriVlvCtrl_D_u8BexvRefriSwitchSt/1

== system ScriptDemo/Create/Model/createMode/After1 ==
  sTmRefriVlvCtrl_X_s32CEXVPosReqIn : Inport  OutDataTypeStr=single
  sTmRefriVlvCtrl_X_s32EEXVPosReqIn : Inport  Port=2  OutDataTypeStr=single
  sTmRefriVlvCtrl_X_s32BEXVPosReqIn : Inport  Port=3  OutDataTypeStr=single
  yTmRefriVlvCtrl_B_HpcCexvMovEnableIn : Inport  Port=4  OutDataTypeStr=boolean
  sTmRefriVlvCtrl_Z_u8CEXVInitStateIn : Inport  Port=5  OutDataTypeStr=uint8
  yTmRefriVlvCtrl_B_CexvCalibReqIn : Inport  Port=6  OutDataTypeStr=boolean
  yTmRefriVlvCtrl_B_HpcEexvMovEnableIn : Inport  Port=7  OutDataTypeStr=boolean
  sTmRefriVlvCtrl_Z_u8EEXVInitStateIn : Inport  Port=8  OutDataTypeStr=uint8
  yTmRefriVlvCtrl_B_EexvCalibReqIn : Inport  Port=9  OutDataTypeStr=boolean
  yTmRefriVlvCtrl_B_HpcBexvMovEnableIn : Inport  Port=10  OutDataTypeStr=boolean
  sTmRefriVlvCtrl_Z_u8BEXVInitStateIn : Inport  Port=11  OutDataTypeStr=uint8
  yTmRefriVlvCtrl_B_BexvCalibReqIn : Inport  Port=12  OutDataTypeStr=boolean
  sTmRefriVlvCtrl_X_s32SM3BexvMaxPosIn : Inport  Port=13  OutDataTypeStr=single
  yTmRefriVlvCtrl_B_EvapBattTLimBexvEnaIn : Inport  Port=14  OutDataTypeStr=boolean
  sTmRefriVlvCtrl_D_u8EexvRefriSwitchStIn : Inport  Port=15  OutDataTypeStr=uint8
  sTmRefriVlvCtrl_D_u8CexvRefriSwitchStIn : Inport  Port=16  OutDataTypeStr=uint8
  sTmRefriVlvCtrl_D_u8BexvRefriSwitchStIn : Inport  Port=17  OutDataTypeStr=uint8
  After1 : Subsystem
  sTmRefriVlvCtrl_X_s32CEXVPosReq : Outport  OutDataTypeStr=single
  sTmRefriVlvCtrl_X_s32EEXVPosReq : Outport  Port=2  OutDataTypeStr=single
  sTmRefriVlvCtrl_X_s32BEXVPosReq : Outport  Port=3  OutDataTypeStr=single
  yTmRefriVlvCtrl_B_HpcCexvMovEnable : Outport  Port=4  OutDataTypeStr=boolean
  sTmRefriVlvCtrl_Z_u8CEXVInitState : Outport  Port=5  OutDataTypeStr=uint8
  yTmRefriVlvCtrl_B_CexvCalibReq : Outport  Port=6  OutDataTypeStr=boolean
  yTmRefriVlvCtrl_B_HpcEexvMovEnable : Outport  Port=7  OutDataTypeStr=boolean
  sTmRefriVlvCtrl_Z_u8EEXVInitState : Outport  Port=8  OutDataTypeStr=uint8
  yTmRefriVlvCtrl_B_EexvCalibReq : Outport  Port=9  OutDataTypeStr=boolean
  yTmRefriVlvCtrl_B_HpcBexvMovEnable : Outport  Port=10  OutDataTypeStr=boolean
  sTmRefriVlvCtrl_Z_u8BEXVInitState : Outport  Port=11  OutDataTypeStr=uint8
  yTmRefriVlvCtrl_B_BexvCalibReq : Outport  Port=12  OutDataTypeStr=boolean
  sTmRefriVlvCtrl_X_s32SM3BexvMaxPos : Outport  Port=13  OutDataTypeStr=single
  yTmRefriVlvCtrl_B_EvapBattTLimBexvEna : Outport  Port=14  OutDataTypeStr=boolean
  sTmRefriVlvCtrl_D_u8EexvRefriSwitchSt : Outport  Port=15  OutDataTypeStr=uint8
  sTmRefriVlvCtrl_D_u8CexvRefriSwitchSt : Outport  Port=16  OutDataTypeStr=uint8
  sTmRefriVlvCtrl_D_u8BexvRefriSwitchSt : Outport  Port=17  OutDataTypeStr=uint8
  wires:
  sTmRefriVlvCtrl_X_s32SM3BexvMaxPosIn/1 -> After1/13(sTmRefriVlvCtrl_X_s32SM3BexvMaxPosIn)
  After1/12(yTmRefriVlvCtrl_B_BexvCalibReq) -> yTmRefriVlvCtrl_B_BexvCalibReq/1  "yTmRefriVlvCtrl_B_BexvCalibReq"
  After1/8(sTmRefriVlvCtrl_Z_u8EEXVInitState) -> sTmRefriVlvCtrl_Z_u8EEXVInitState/1  "sTmRefriVlvCtrl_Z_u8EEXVInitState"
  After1/10(yTmRefriVlvCtrl_B_HpcBexvMovEnable) -> yTmRefriVlvCtrl_B_HpcBexvMovEnable/1  "yTmRefriVlvCtrl_B_HpcBexvMovEnable"
  sTmRefriVlvCtrl_Z_u8BEXVInitStateIn/1 -> After1/11(sTmRefriVlvCtrl_Z_u8BEXVInitStateIn)
  sTmRefriVlvCtrl_Z_u8EEXVInitStateIn/1 -> After1/8(sTmRefriVlvCtrl_Z_u8EEXVInitStateIn)
  After1/16(sTmRefriVlvCtrl_D_u8CexvRefriSwitchSt) -> sTmRefriVlvCtrl_D_u8CexvRefriSwitchSt/1  "sTmRefriVlvCtrl_D_u8CexvRefriSwitchSt"
  After1/3(sTmRefriVlvCtrl_X_s32BEXVPosReq) -> sTmRefriVlvCtrl_X_s32BEXVPosReq/1  "sTmRefriVlvCtrl_X_s32BEXVPosReq"
  After1/6(yTmRefriVlvCtrl_B_CexvCalibReq) -> yTmRefriVlvCtrl_B_CexvCalibReq/1  "yTmRefriVlvCtrl_B_CexvCalibReq"
  After1/5(sTmRefriVlvCtrl_Z_u8CEXVInitState) -> sTmRefriVlvCtrl_Z_u8CEXVInitState/1  "sTmRefriVlvCtrl_Z_u8CEXVInitState"
  After1/7(yTmRefriVlvCtrl_B_HpcEexvMovEnable) -> yTmRefriVlvCtrl_B_HpcEexvMovEnable/1  "yTmRefriVlvCtrl_B_HpcEexvMovEnable"
  sTmRefriVlvCtrl_Z_u8CEXVInitStateIn/1 -> After1/5(sTmRefriVlvCtrl_Z_u8CEXVInitStateIn)
  After1/9(yTmRefriVlvCtrl_B_EexvCalibReq) -> yTmRefriVlvCtrl_B_EexvCalibReq/1  "yTmRefriVlvCtrl_B_EexvCalibReq"
  After1/13(sTmRefriVlvCtrl_X_s32SM3BexvMaxPos) -> sTmRefriVlvCtrl_X_s32SM3BexvMaxPos/1  "sTmRefriVlvCtrl_X_s32SM3BexvMaxPos"
  sTmRefriVlvCtrl_D_u8EexvRefriSwitchStIn/1 -> After1/15(sTmRefriVlvCtrl_D_u8EexvRefriSwitchStIn)
  After1/11(sTmRefriVlvCtrl_Z_u8BEXVInitState) -> sTmRefriVlvCtrl_Z_u8BEXVInitState/1  "sTmRefriVlvCtrl_Z_u8BEXVInitState"
  After1/14(yTmRefriVlvCtrl_B_EvapBattTLimBexvEna) -> yTmRefriVlvCtrl_B_EvapBattTLimBexvEna/1  "yTmRefriVlvCtrl_B_EvapBattTLimBexvEna"
  After1/15(sTmRefriVlvCtrl_D_u8EexvRefriSwitchSt) -> sTmRefriVlvCtrl_D_u8EexvRefriSwitchSt/1  "sTmRefriVlvCtrl_D_u8EexvRefriSwitchSt"
  sTmRefriVlvCtrl_X_s32CEXVPosReqIn/1 -> After1/1(sTmRefriVlvCtrl_X_s32CEXVPosReqIn)
  yTmRefriVlvCtrl_B_HpcCexvMovEnableIn/1 -> After1/4(yTmRefriVlvCtrl_B_HpcCexvMovEnableIn)
  After1/17(sTmRefriVlvCtrl_D_u8BexvRefriSwitchSt) -> sTmRefriVlvCtrl_D_u8BexvRefriSwitchSt/1  "sTmRefriVlvCtrl_D_u8BexvRefriSwitchSt"
  sTmRefriVlvCtrl_D_u8CexvRefriSwitchStIn/1 -> After1/16(sTmRefriVlvCtrl_D_u8CexvRefriSwitchStIn)
  yTmRefriVlvCtrl_B_EvapBattTLimBexvEnaIn/1 -> After1/14(yTmRefriVlvCtrl_B_EvapBattTLimBexvEnaIn)
  yTmRefriVlvCtrl_B_HpcBexvMovEnableIn/1 -> After1/10(yTmRefriVlvCtrl_B_HpcBexvMovEnableIn)
  yTmRefriVlvCtrl_B_HpcEexvMovEnableIn/1 -> After1/7(yTmRefriVlvCtrl_B_HpcEexvMovEnableIn)
  yTmRefriVlvCtrl_B_BexvCalibReqIn/1 -> After1/12(yTmRefriVlvCtrl_B_BexvCalibReqIn)
  After1/4(yTmRefriVlvCtrl_B_HpcCexvMovEnable) -> yTmRefriVlvCtrl_B_HpcCexvMovEnable/1  "yTmRefriVlvCtrl_B_HpcCexvMovEnable"
  After1/2(sTmRefriVlvCtrl_X_s32EEXVPosReq) -> sTmRefriVlvCtrl_X_s32EEXVPosReq/1  "sTmRefriVlvCtrl_X_s32EEXVPosReq"
  sTmRefriVlvCtrl_X_s32BEXVPosReqIn/1 -> After1/3(sTmRefriVlvCtrl_X_s32BEXVPosReqIn)
  sTmRefriVlvCtrl_D_u8BexvRefriSwitchStIn/1 -> After1/17(sTmRefriVlvCtrl_D_u8BexvRefriSwitchStIn)
  After1/1(sTmRefriVlvCtrl_X_s32CEXVPosReq) -> sTmRefriVlvCtrl_X_s32CEXVPosReq/1  "sTmRefriVlvCtrl_X_s32CEXVPosReq"
  yTmRefriVlvCtrl_B_EexvCalibReqIn/1 -> After1/9(yTmRefriVlvCtrl_B_EexvCalibReqIn)
  sTmRefriVlvCtrl_X_s32EEXVPosReqIn/1 -> After1/2(sTmRefriVlvCtrl_X_s32EEXVPosReqIn)
  yTmRefriVlvCtrl_B_CexvCalibReqIn/1 -> After1/6(yTmRefriVlvCtrl_B_CexvCalibReqIn)

== system ScriptDemo/Create/Model/createMode/After2 ==
  note: createMode(gcb, ...
      | 'inType' , 'from' , ... % 可选参数 port, ground, from, const, none
      | 'outType' , 'port' , ... % 可选参数 port, term, goto, disp, none
      | 'suffixStr' , 'In' , ...
      | ... % 创建 ports 相关配置
      | 'add' , 'None' , ... % 可选参数 blockType, None, etc：SignalConversion
      | ... % 创建 goto from 相关配置
      | 'bkHalfLength' , 125, ...
      | ... % 创建 信号解析 相关配置
      | 'isEnableIn' ,false, ...
      | 'isEnableOut' ,true, ...
      | 'resoveValue' ,true, ...
      | 'logValue' ,false, ...
      | 'testValue' ,false, ...
      | 'dispName' , false ...
      | )
  After1 : Subsystem
  sTmRefriVlvCtrl_X_s32CEXVPosReq : Outport  OutDataTypeStr=single
  sTmRefriVlvCtrl_X_s32EEXVPosReq : Outport  Port=2  OutDataTypeStr=single
  sTmRefriVlvCtrl_X_s32BEXVPosReq : Outport  Port=3  OutDataTypeStr=single
  yTmRefriVlvCtrl_B_HpcCexvMovEnable : Outport  Port=4  OutDataTypeStr=boolean
  sTmRefriVlvCtrl_Z_u8CEXVInitState : Outport  Port=5  OutDataTypeStr=uint8
  yTmRefriVlvCtrl_B_CexvCalibReq : Outport  Port=6  OutDataTypeStr=boolean
  yTmRefriVlvCtrl_B_HpcEexvMovEnable : Outport  Port=7  OutDataTypeStr=boolean
  sTmRefriVlvCtrl_Z_u8EEXVInitState : Outport  Port=8  OutDataTypeStr=uint8
  yTmRefriVlvCtrl_B_EexvCalibReq : Outport  Port=9  OutDataTypeStr=boolean
  yTmRefriVlvCtrl_B_HpcBexvMovEnable : Outport  Port=10  OutDataTypeStr=boolean
  sTmRefriVlvCtrl_Z_u8BEXVInitState : Outport  Port=11  OutDataTypeStr=uint8
  yTmRefriVlvCtrl_B_BexvCalibReq : Outport  Port=12  OutDataTypeStr=boolean
  sTmRefriVlvCtrl_X_s32SM3BexvMaxPos : Outport  Port=13  OutDataTypeStr=single
  yTmRefriVlvCtrl_B_EvapBattTLimBexvEna : Outport  Port=14  OutDataTypeStr=boolean
  sTmRefriVlvCtrl_D_u8EexvRefriSwitchSt : Outport  Port=15  OutDataTypeStr=uint8
  sTmRefriVlvCtrl_D_u8CexvRefriSwitchSt : Outport  Port=16  OutDataTypeStr=uint8
  sTmRefriVlvCtrl_D_u8BexvRefriSwitchSt : Outport  Port=17  OutDataTypeStr=uint8
  wires:
  [sTmRefriVlvCtrl_X_s32CEXVPosReq] -> After1/1(sTmRefriVlvCtrl_X_s32CEXVPosReqIn)
  [sTmRefriVlvCtrl_X_s32EEXVPosReq] -> After1/2(sTmRefriVlvCtrl_X_s32EEXVPosReqIn)
  [sTmRefriVlvCtrl_X_s32BEXVPosReq] -> After1/3(sTmRefriVlvCtrl_X_s32BEXVPosReqIn)
  [yTmRefriVlvCtrl_B_HpcCexvMovEnable] -> After1/4(yTmRefriVlvCtrl_B_HpcCexvMovEnableIn)
  [sTmRefriVlvCtrl_Z_u8CEXVInitState] -> After1/5(sTmRefriVlvCtrl_Z_u8CEXVInitStateIn)
  [yTmRefriVlvCtrl_B_CexvCalibReq] -> After1/6(yTmRefriVlvCtrl_B_CexvCalibReqIn)
  [yTmRefriVlvCtrl_B_HpcEexvMovEnable] -> After1/7(yTmRefriVlvCtrl_B_HpcEexvMovEnableIn)
  [sTmRefriVlvCtrl_Z_u8EEXVInitState] -> After1/8(sTmRefriVlvCtrl_Z_u8EEXVInitStateIn)
  [yTmRefriVlvCtrl_B_EexvCalibReq] -> After1/9(yTmRefriVlvCtrl_B_EexvCalibReqIn)
  [yTmRefriVlvCtrl_B_HpcBexvMovEnable] -> After1/10(yTmRefriVlvCtrl_B_HpcBexvMovEnableIn)
  [sTmRefriVlvCtrl_Z_u8BEXVInitState] -> After1/11(sTmRefriVlvCtrl_Z_u8BEXVInitStateIn)
  [yTmRefriVlvCtrl_B_BexvCalibReq] -> After1/12(yTmRefriVlvCtrl_B_BexvCalibReqIn)
  [sTmRefriVlvCtrl_X_s32SM3BexvMaxPos] -> After1/13(sTmRefriVlvCtrl_X_s32SM3BexvMaxPosIn)
  [yTmRefriVlvCtrl_B_EvapBattTLimBexvEna] -> After1/14(yTmRefriVlvCtrl_B_EvapBattTLimBexvEnaIn)
  [sTmRefriVlvCtrl_D_u8EexvRefriSwitchSt] -> After1/15(sTmRefriVlvCtrl_D_u8EexvRefriSwitchStIn)
  [sTmRefriVlvCtrl_D_u8CexvRefriSwitchSt] -> After1/16(sTmRefriVlvCtrl_D_u8CexvRefriSwitchStIn)
  [sTmRefriVlvCtrl_D_u8BexvRefriSwitchSt] -> After1/17(sTmRefriVlvCtrl_D_u8BexvRefriSwitchStIn)
  After1/1(sTmRefriVlvCtrl_X_s32CEXVPosReq) -> sTmRefriVlvCtrl_X_s32CEXVPosReq/1  "sTmRefriVlvCtrl_X_s32CEXVPosReq"
  After1/2(sTmRefriVlvCtrl_X_s32EEXVPosReq) -> sTmRefriVlvCtrl_X_s32EEXVPosReq/1  "sTmRefriVlvCtrl_X_s32EEXVPosReq"
  After1/3(sTmRefriVlvCtrl_X_s32BEXVPosReq) -> sTmRefriVlvCtrl_X_s32BEXVPosReq/1  "sTmRefriVlvCtrl_X_s32BEXVPosReq"
  After1/4(yTmRefriVlvCtrl_B_HpcCexvMovEnable) -> yTmRefriVlvCtrl_B_HpcCexvMovEnable/1  "yTmRefriVlvCtrl_B_HpcCexvMovEnable"
  After1/5(sTmRefriVlvCtrl_Z_u8CEXVInitState) -> sTmRefriVlvCtrl_Z_u8CEXVInitState/1  "sTmRefriVlvCtrl_Z_u8CEXVInitState"
  After1/6(yTmRefriVlvCtrl_B_CexvCalibReq) -> yTmRefriVlvCtrl_B_CexvCalibReq/1  "yTmRefriVlvCtrl_B_CexvCalibReq"
  After1/7(yTmRefriVlvCtrl_B_HpcEexvMovEnable) -> yTmRefriVlvCtrl_B_HpcEexvMovEnable/1  "yTmRefriVlvCtrl_B_HpcEexvMovEnable"
  After1/8(sTmRefriVlvCtrl_Z_u8EEXVInitState) -> sTmRefriVlvCtrl_Z_u8EEXVInitState/1  "sTmRefriVlvCtrl_Z_u8EEXVInitState"
  After1/9(yTmRefriVlvCtrl_B_EexvCalibReq) -> yTmRefriVlvCtrl_B_EexvCalibReq/1  "yTmRefriVlvCtrl_B_EexvCalibReq"
  After1/10(yTmRefriVlvCtrl_B_HpcBexvMovEnable) -> yTmRefriVlvCtrl_B_HpcBexvMovEnable/1  "yTmRefriVlvCtrl_B_HpcBexvMovEnable"
  After1/11(sTmRefriVlvCtrl_Z_u8BEXVInitState) -> sTmRefriVlvCtrl_Z_u8BEXVInitState/1  "sTmRefriVlvCtrl_Z_u8BEXVInitState"
  After1/12(yTmRefriVlvCtrl_B_BexvCalibReq) -> yTmRefriVlvCtrl_B_BexvCalibReq/1  "yTmRefriVlvCtrl_B_BexvCalibReq"
  After1/13(sTmRefriVlvCtrl_X_s32SM3BexvMaxPos) -> sTmRefriVlvCtrl_X_s32SM3BexvMaxPos/1  "sTmRefriVlvCtrl_X_s32SM3BexvMaxPos"
  After1/14(yTmRefriVlvCtrl_B_EvapBattTLimBexvEna) -> yTmRefriVlvCtrl_B_EvapBattTLimBexvEna/1  "yTmRefriVlvCtrl_B_EvapBattTLimBexvEna"
  After1/15(sTmRefriVlvCtrl_D_u8EexvRefriSwitchSt) -> sTmRefriVlvCtrl_D_u8EexvRefriSwitchSt/1  "sTmRefriVlvCtrl_D_u8EexvRefriSwitchSt"
  After1/16(sTmRefriVlvCtrl_D_u8CexvRefriSwitchSt) -> sTmRefriVlvCtrl_D_u8CexvRefriSwitchSt/1  "sTmRefriVlvCtrl_D_u8CexvRefriSwitchSt"
  After1/17(sTmRefriVlvCtrl_D_u8BexvRefriSwitchSt) -> sTmRefriVlvCtrl_D_u8BexvRefriSwitchSt/1  "sTmRefriVlvCtrl_D_u8BexvRefriSwitchSt"

== system ScriptDemo/Create/Model/createMode/After3 ==
  note: createMode(gcb, ...
      | 'inType' , 'const' , ... % 可选参数 port, ground, from, const, none
      | 'outType' , 'disp' , ... % 可选参数 port, term, goto, disp, none
      | 'suffixStr' , 'In' , ...
      | ... % 创建 ports 相关配置
      | 'add' , 'None' , ... % 可选参数 blockType, None, etc：SignalConversion
      | ... % 创建 goto from 相关配置
      | 'bkHalfLength' , 125, ...
      | ... % 创建 信号解析 相关配置
      | 'isEnableIn' ,false, ...
      | 'isEnableOut' ,true, ...
      | 'resoveValue' ,false, ...
      | 'logValue' ,true, ...
      | 'testValue' ,false, ...
      | 'dispName' , false ...
      | )
  After1 : Subsystem
  Constant{,1..2,12} (4 alike) : Constant  Value=0  OutDataTypeStr=single
  Constant{4,7,10,14..16} (6 alike) : Constant  Value=0  OutDataTypeStr=uint8
  Constant{3,5..6,8..9,11,13} (7 alike) : Constant  Value=0  OutDataTypeStr=boolean
  Display{,1..16} (17 alike) : Display
  wires:
  Constant/1 -> After1/1(sTmRefriVlvCtrl_X_s32CEXVPosReqIn)
  Constant1/1 -> After1/2(sTmRefriVlvCtrl_X_s32EEXVPosReqIn)
  Constant2/1 -> After1/3(sTmRefriVlvCtrl_X_s32BEXVPosReqIn)
  Constant3/1 -> After1/4(yTmRefriVlvCtrl_B_HpcCexvMovEnableIn)
  Constant4/1 -> After1/5(sTmRefriVlvCtrl_Z_u8CEXVInitStateIn)
  Constant5/1 -> After1/6(yTmRefriVlvCtrl_B_CexvCalibReqIn)
  Constant6/1 -> After1/7(yTmRefriVlvCtrl_B_HpcEexvMovEnableIn)
  Constant7/1 -> After1/8(sTmRefriVlvCtrl_Z_u8EEXVInitStateIn)
  Constant8/1 -> After1/9(yTmRefriVlvCtrl_B_EexvCalibReqIn)
  Constant9/1 -> After1/10(yTmRefriVlvCtrl_B_HpcBexvMovEnableIn)
  Constant10/1 -> After1/11(sTmRefriVlvCtrl_Z_u8BEXVInitStateIn)
  Constant11/1 -> After1/12(yTmRefriVlvCtrl_B_BexvCalibReqIn)
  Constant12/1 -> After1/13(sTmRefriVlvCtrl_X_s32SM3BexvMaxPosIn)
  Constant13/1 -> After1/14(yTmRefriVlvCtrl_B_EvapBattTLimBexvEnaIn)
  Constant14/1 -> After1/15(sTmRefriVlvCtrl_D_u8EexvRefriSwitchStIn)
  Constant15/1 -> After1/16(sTmRefriVlvCtrl_D_u8CexvRefriSwitchStIn)
  Constant16/1 -> After1/17(sTmRefriVlvCtrl_D_u8BexvRefriSwitchStIn)
  After1/1(sTmRefriVlvCtrl_X_s32CEXVPosReq) -> Display/1
  After1/2(sTmRefriVlvCtrl_X_s32EEXVPosReq) -> Display1/1
  After1/3(sTmRefriVlvCtrl_X_s32BEXVPosReq) -> Display2/1
  After1/4(yTmRefriVlvCtrl_B_HpcCexvMovEnable) -> Display3/1
  After1/5(sTmRefriVlvCtrl_Z_u8CEXVInitState) -> Display4/1
  After1/6(yTmRefriVlvCtrl_B_CexvCalibReq) -> Display5/1
  After1/7(yTmRefriVlvCtrl_B_HpcEexvMovEnable) -> Display6/1
  After1/8(sTmRefriVlvCtrl_Z_u8EEXVInitState) -> Display7/1
  After1/9(yTmRefriVlvCtrl_B_EexvCalibReq) -> Display8/1
  After1/10(yTmRefriVlvCtrl_B_HpcBexvMovEnable) -> Display9/1
  After1/11(sTmRefriVlvCtrl_Z_u8BEXVInitState) -> Display10/1
  After1/12(yTmRefriVlvCtrl_B_BexvCalibReq) -> Display11/1
  After1/13(sTmRefriVlvCtrl_X_s32SM3BexvMaxPos) -> Display12/1
  After1/14(yTmRefriVlvCtrl_B_EvapBattTLimBexvEna) -> Display13/1
  After1/15(sTmRefriVlvCtrl_D_u8EexvRefriSwitchSt) -> Display14/1
  After1/16(sTmRefriVlvCtrl_D_u8CexvRefriSwitchSt) -> Display15/1
  After1/17(sTmRefriVlvCtrl_D_u8BexvRefriSwitchSt) -> Display16/1

== system ScriptDemo/Create/Model/createMode/After4 ==
  note: createMode(gcb, ...
      | 'inType' , 'ground' , ... % 可选参数 port, ground, from, const, none
      | 'outType' , 'term' , ... % 可选参数 port, term, goto, disp, none
      | 'suffixStr' , 'In' , ...
      | ... % 创建 ports 相关配置
      | 'add' , 'None' , ... % 可选参数 blockType, None, etc：SignalConversion
      | ... % 创建 goto from 相关配置
      | 'bkHalfLength' , 125, ...
      | ... % 创建 信号解析 相关配置
      | 'isEnableIn' ,true, ...
      | 'isEnableOut' ,true, ...
      | 'resoveValue' ,false, ...
      | 'logValue' ,false, ...
      | 'testValue' ,false, ...
      | 'dispName' , false ...
      | )
  After1 : Subsystem
  Ground{,1..16} (17 alike) : Ground
  Terminator{,1..16} (17 alike) : Terminator
  wires:
  Ground/1 -> After1/1(sTmRefriVlvCtrl_X_s32CEXVPosReqIn)
  Ground1/1 -> After1/2(sTmRefriVlvCtrl_X_s32EEXVPosReqIn)
  Ground2/1 -> After1/3(sTmRefriVlvCtrl_X_s32BEXVPosReqIn)
  Ground3/1 -> After1/4(yTmRefriVlvCtrl_B_HpcCexvMovEnableIn)
  Ground4/1 -> After1/5(sTmRefriVlvCtrl_Z_u8CEXVInitStateIn)
  Ground5/1 -> After1/6(yTmRefriVlvCtrl_B_CexvCalibReqIn)
  Ground6/1 -> After1/7(yTmRefriVlvCtrl_B_HpcEexvMovEnableIn)
  Ground7/1 -> After1/8(sTmRefriVlvCtrl_Z_u8EEXVInitStateIn)
  Ground8/1 -> After1/9(yTmRefriVlvCtrl_B_EexvCalibReqIn)
  Ground9/1 -> After1/10(yTmRefriVlvCtrl_B_HpcBexvMovEnableIn)
  Ground10/1 -> After1/11(sTmRefriVlvCtrl_Z_u8BEXVInitStateIn)
  Ground11/1 -> After1/12(yTmRefriVlvCtrl_B_BexvCalibReqIn)
  Ground12/1 -> After1/13(sTmRefriVlvCtrl_X_s32SM3BexvMaxPosIn)
  Ground13/1 -> After1/14(yTmRefriVlvCtrl_B_EvapBattTLimBexvEnaIn)
  Ground14/1 -> After1/15(sTmRefriVlvCtrl_D_u8EexvRefriSwitchStIn)
  Ground15/1 -> After1/16(sTmRefriVlvCtrl_D_u8CexvRefriSwitchStIn)
  Ground16/1 -> After1/17(sTmRefriVlvCtrl_D_u8BexvRefriSwitchStIn)
  After1/1(sTmRefriVlvCtrl_X_s32CEXVPosReq) -> Terminator/1
  After1/2(sTmRefriVlvCtrl_X_s32EEXVPosReq) -> Terminator1/1
  After1/3(sTmRefriVlvCtrl_X_s32BEXVPosReq) -> Terminator2/1
  After1/4(yTmRefriVlvCtrl_B_HpcCexvMovEnable) -> Terminator3/1
  After1/5(sTmRefriVlvCtrl_Z_u8CEXVInitState) -> Terminator4/1
  After1/6(yTmRefriVlvCtrl_B_CexvCalibReq) -> Terminator5/1
  After1/7(yTmRefriVlvCtrl_B_HpcEexvMovEnable) -> Terminator6/1
  After1/8(sTmRefriVlvCtrl_Z_u8EEXVInitState) -> Terminator7/1
  After1/9(yTmRefriVlvCtrl_B_EexvCalibReq) -> Terminator8/1
  After1/10(yTmRefriVlvCtrl_B_HpcBexvMovEnable) -> Terminator9/1
  After1/11(sTmRefriVlvCtrl_Z_u8BEXVInitState) -> Terminator10/1
  After1/12(yTmRefriVlvCtrl_B_BexvCalibReq) -> Terminator11/1
  After1/13(sTmRefriVlvCtrl_X_s32SM3BexvMaxPos) -> Terminator12/1
  After1/14(yTmRefriVlvCtrl_B_EvapBattTLimBexvEna) -> Terminator13/1
  After1/15(sTmRefriVlvCtrl_D_u8EexvRefriSwitchSt) -> Terminator14/1
  After1/16(sTmRefriVlvCtrl_D_u8CexvRefriSwitchSt) -> Terminator15/1
  After1/17(sTmRefriVlvCtrl_D_u8BexvRefriSwitchSt) -> Terminator16/1

== system ScriptDemo/Create/Model/createMode/After5 ==
  note: createMode(gcb, ...
      | 'inType' , 'none' , ... % 可选参数 port, ground, from, const, none
      | 'outType' , 'port' , ... % 可选参数 port, term, goto, disp, none
      | 'suffixStr' , '' , ...
      | ... % 创建 ports 相关配置
      | 'add' , 'SignalConversion' , ... % 可选参数 blockType, None, etc：SignalConversion
      | ... % 创建 goto from 相关配置
      | 'bkHalfLength' , 125, ...
      | ... % 创建 信号解析 相关配置
      | 'isEnableIn' ,true, ...
      | 'isEnableOut' ,true, ...
      | 'resoveValue' ,false, ...
      | 'logValue' ,false, ...
      | 'testValue' ,false, ...
      | 'dispName' , false ...
      | )
      |
      | createMode(gcb, ...
      | 'inType' , 'port' , ... % 可选参数 port, ground, from, const, none
      | 'outType' , 'none' , ... % 可选参数 port, term, goto, disp, none
      | 'suffixStr' , '' , ...
      | ... % 创建 ports 相关配置
      | 'add' , 'DataTypeConversion' , ... % 可选参数 blockType, None, etc：SignalConversion DataTypeConversion
      | ... % 创建 goto from 相关配置
      | 'bkHalfLength' , 125, ...
      | ... % 创建 信号解析 相关配置
      | 'isEnableIn' ,true, ...
      | 'isEnableOut' ,true, ...
      | 'resoveValue' ,false, ...
      | 'logValue' ,false, ...
      | 'testValue' ,false, ...
      | 'dispName' , false ...
      | )
  sTmRefriVlvCtrl_X_s32CEXVPosReqIn : Inport  OutDataTypeStr=single
  sTmRefriVlvCtrl_X_s32EEXVPosReqIn : Inport  Port=2  OutDataTypeStr=single
  sTmRefriVlvCtrl_X_s32BEXVPosReqIn : Inport  Port=3  OutDataTypeStr=single
  yTmRefriVlvCtrl_B_HpcCexvMovEnableIn : Inport  Port=4  OutDataTypeStr=boolean
  sTmRefriVlvCtrl_Z_u8CEXVInitStateIn : Inport  Port=5  OutDataTypeStr=uint8
  yTmRefriVlvCtrl_B_CexvCalibReqIn : Inport  Port=6  OutDataTypeStr=boolean
  yTmRefriVlvCtrl_B_HpcEexvMovEnableIn : Inport  Port=7  OutDataTypeStr=boolean
  sTmRefriVlvCtrl_Z_u8EEXVInitStateIn : Inport  Port=8  OutDataTypeStr=uint8
  yTmRefriVlvCtrl_B_EexvCalibReqIn : Inport  Port=9  OutDataTypeStr=boolean
  yTmRefriVlvCtrl_B_HpcBexvMovEnableIn : Inport  Port=10  OutDataTypeStr=boolean
  sTmRefriVlvCtrl_Z_u8BEXVInitStateIn : Inport  Port=11  OutDataTypeStr=uint8
  yTmRefriVlvCtrl_B_BexvCalibReqIn : Inport  Port=12  OutDataTypeStr=boolean
  sTmRefriVlvCtrl_X_s32SM3BexvMaxPosIn : Inport  Port=13  OutDataTypeStr=single
  yTmRefriVlvCtrl_B_EvapBattTLimBexvEnaIn : Inport  Port=14  OutDataTypeStr=boolean
  sTmRefriVlvCtrl_D_u8EexvRefriSwitchStIn : Inport  Port=15  OutDataTypeStr=uint8
  sTmRefriVlvCtrl_D_u8CexvRefriSwitchStIn : Inport  Port=16  OutDataTypeStr=uint8
  sTmRefriVlvCtrl_D_u8BexvRefriSwitchStIn : Inport  Port=17  OutDataTypeStr=uint8
  After1 : Subsystem
  sigCov{,1..16} (17 alike) : SignalConversion  OverrideOpt=off
  sigCov{17..33} (17 alike) : DataTypeConversion
  sTmRefriVlvCtrl_X_s32CEXVPosReq : Outport  OutDataTypeStr=single
  sTmRefriVlvCtrl_X_s32EEXVPosReq : Outport  Port=2  OutDataTypeStr=single
  sTmRefriVlvCtrl_X_s32BEXVPosReq : Outport  Port=3  OutDataTypeStr=single
  yTmRefriVlvCtrl_B_HpcCexvMovEnable : Outport  Port=4  OutDataTypeStr=boolean
  sTmRefriVlvCtrl_Z_u8CEXVInitState : Outport  Port=5  OutDataTypeStr=uint8
  yTmRefriVlvCtrl_B_CexvCalibReq : Outport  Port=6  OutDataTypeStr=boolean
  yTmRefriVlvCtrl_B_HpcEexvMovEnable : Outport  Port=7  OutDataTypeStr=boolean
  sTmRefriVlvCtrl_Z_u8EEXVInitState : Outport  Port=8  OutDataTypeStr=uint8
  yTmRefriVlvCtrl_B_EexvCalibReq : Outport  Port=9  OutDataTypeStr=boolean
  yTmRefriVlvCtrl_B_HpcBexvMovEnable : Outport  Port=10  OutDataTypeStr=boolean
  sTmRefriVlvCtrl_Z_u8BEXVInitState : Outport  Port=11  OutDataTypeStr=uint8
  yTmRefriVlvCtrl_B_BexvCalibReq : Outport  Port=12  OutDataTypeStr=boolean
  sTmRefriVlvCtrl_X_s32SM3BexvMaxPos : Outport  Port=13  OutDataTypeStr=single
  yTmRefriVlvCtrl_B_EvapBattTLimBexvEna : Outport  Port=14  OutDataTypeStr=boolean
  sTmRefriVlvCtrl_D_u8EexvRefriSwitchSt : Outport  Port=15  OutDataTypeStr=uint8
  sTmRefriVlvCtrl_D_u8CexvRefriSwitchSt : Outport  Port=16  OutDataTypeStr=uint8
  sTmRefriVlvCtrl_D_u8BexvRefriSwitchSt : Outport  Port=17  OutDataTypeStr=uint8
  wires:
  After1/1(sTmRefriVlvCtrl_X_s32CEXVPosReq) -> sigCov/1
  sigCov/1 -> sTmRefriVlvCtrl_X_s32CEXVPosReq/1
  After1/2(sTmRefriVlvCtrl_X_s32EEXVPosReq) -> sigCov1/1
  sigCov1/1 -> sTmRefriVlvCtrl_X_s32EEXVPosReq/1
  After1/3(sTmRefriVlvCtrl_X_s32BEXVPosReq) -> sigCov2/1
  sigCov2/1 -> sTmRefriVlvCtrl_X_s32BEXVPosReq/1
  After1/4(yTmRefriVlvCtrl_B_HpcCexvMovEnable) -> sigCov3/1
  sigCov3/1 -> yTmRefriVlvCtrl_B_HpcCexvMovEnable/1
  After1/5(sTmRefriVlvCtrl_Z_u8CEXVInitState) -> sigCov4/1
  sigCov4/1 -> sTmRefriVlvCtrl_Z_u8CEXVInitState/1
  After1/6(yTmRefriVlvCtrl_B_CexvCalibReq) -> sigCov5/1
  sigCov5/1 -> yTmRefriVlvCtrl_B_CexvCalibReq/1
  After1/7(yTmRefriVlvCtrl_B_HpcEexvMovEnable) -> sigCov6/1
  sigCov6/1 -> yTmRefriVlvCtrl_B_HpcEexvMovEnable/1
  After1/8(sTmRefriVlvCtrl_Z_u8EEXVInitState) -> sigCov7/1
  sigCov7/1 -> sTmRefriVlvCtrl_Z_u8EEXVInitState/1
  After1/9(yTmRefriVlvCtrl_B_EexvCalibReq) -> sigCov8/1
  sigCov8/1 -> yTmRefriVlvCtrl_B_EexvCalibReq/1
  After1/10(yTmRefriVlvCtrl_B_HpcBexvMovEnable) -> sigCov9/1
  sigCov9/1 -> yTmRefriVlvCtrl_B_HpcBexvMovEnable/1
  After1/11(sTmRefriVlvCtrl_Z_u8BEXVInitState) -> sigCov10/1
  sigCov10/1 -> sTmRefriVlvCtrl_Z_u8BEXVInitState/1
  After1/12(yTmRefriVlvCtrl_B_BexvCalibReq) -> sigCov11/1
  sigCov11/1 -> yTmRefriVlvCtrl_B_BexvCalibReq/1
  After1/13(sTmRefriVlvCtrl_X_s32SM3BexvMaxPos) -> sigCov12/1
  sigCov12/1 -> sTmRefriVlvCtrl_X_s32SM3BexvMaxPos/1
  After1/14(yTmRefriVlvCtrl_B_EvapBattTLimBexvEna) -> sigCov13/1
  sigCov13/1 -> yTmRefriVlvCtrl_B_EvapBattTLimBexvEna/1
  After1/15(sTmRefriVlvCtrl_D_u8EexvRefriSwitchSt) -> sigCov14/1
  sigCov14/1 -> sTmRefriVlvCtrl_D_u8EexvRefriSwitchSt/1
  After1/16(sTmRefriVlvCtrl_D_u8CexvRefriSwitchSt) -> sigCov15/1
  sigCov15/1 -> sTmRefriVlvCtrl_D_u8CexvRefriSwitchSt/1
  After1/17(sTmRefriVlvCtrl_D_u8BexvRefriSwitchSt) -> sigCov16/1
  sigCov16/1 -> sTmRefriVlvCtrl_D_u8BexvRefriSwitchSt/1
  sTmRefriVlvCtrl_X_s32CEXVPosReqIn/1 -> sigCov17/1
  sigCov17/1 -> After1/1(sTmRefriVlvCtrl_X_s32CEXVPosReqIn)
  sTmRefriVlvCtrl_X_s32EEXVPosReqIn/1 -> sigCov18/1
  sigCov18/1 -> After1/2(sTmRefriVlvCtrl_X_s32EEXVPosReqIn)
  sTmRefriVlvCtrl_X_s32BEXVPosReqIn/1 -> sigCov19/1
  sigCov19/1 -> After1/3(sTmRefriVlvCtrl_X_s32BEXVPosReqIn)
  yTmRefriVlvCtrl_B_HpcCexvMovEnableIn/1 -> sigCov20/1
  sigCov20/1 -> After1/4(yTmRefriVlvCtrl_B_HpcCexvMovEnableIn)
  sTmRefriVlvCtrl_Z_u8CEXVInitStateIn/1 -> sigCov21/1
  sigCov21/1 -> After1/5(sTmRefriVlvCtrl_Z_u8CEXVInitStateIn)
  yTmRefriVlvCtrl_B_CexvCalibReqIn/1 -> sigCov22/1
  sigCov22/1 -> After1/6(yTmRefriVlvCtrl_B_CexvCalibReqIn)
  yTmRefriVlvCtrl_B_HpcEexvMovEnableIn/1 -> sigCov23/1
  sigCov23/1 -> After1/7(yTmRefriVlvCtrl_B_HpcEexvMovEnableIn)
  sTmRefriVlvCtrl_Z_u8EEXVInitStateIn/1 -> sigCov24/1
  sigCov24/1 -> After1/8(sTmRefriVlvCtrl_Z_u8EEXVInitStateIn)
  yTmRefriVlvCtrl_B_EexvCalibReqIn/1 -> sigCov25/1
  sigCov25/1 -> After1/9(yTmRefriVlvCtrl_B_EexvCalibReqIn)
  yTmRefriVlvCtrl_B_HpcBexvMovEnableIn/1 -> sigCov26/1
  sigCov26/1 -> After1/10(yTmRefriVlvCtrl_B_HpcBexvMovEnableIn)
  sTmRefriVlvCtrl_Z_u8BEXVInitStateIn/1 -> sigCov27/1
  sigCov27/1 -> After1/11(sTmRefriVlvCtrl_Z_u8BEXVInitStateIn)
  yTmRefriVlvCtrl_B_BexvCalibReqIn/1 -> sigCov28/1
  sigCov28/1 -> After1/12(yTmRefriVlvCtrl_B_BexvCalibReqIn)
  sTmRefriVlvCtrl_X_s32SM3BexvMaxPosIn/1 -> sigCov29/1
  sigCov29/1 -> After1/13(sTmRefriVlvCtrl_X_s32SM3BexvMaxPosIn)
  yTmRefriVlvCtrl_B_EvapBattTLimBexvEnaIn/1 -> sigCov30/1
  sigCov30/1 -> After1/14(yTmRefriVlvCtrl_B_EvapBattTLimBexvEnaIn)
  sTmRefriVlvCtrl_D_u8EexvRefriSwitchStIn/1 -> sigCov31/1
  sigCov31/1 -> After1/15(sTmRefriVlvCtrl_D_u8EexvRefriSwitchStIn)
  sTmRefriVlvCtrl_D_u8CexvRefriSwitchStIn/1 -> sigCov32/1
  sigCov32/1 -> After1/16(sTmRefriVlvCtrl_D_u8CexvRefriSwitchStIn)
  sTmRefriVlvCtrl_D_u8BexvRefriSwitchStIn/1 -> sigCov33/1
  sigCov33/1 -> After1/17(sTmRefriVlvCtrl_D_u8BexvRefriSwitchStIn)
